simulink model "HEV_Ctrl_V1_1"  (R2018a)
settings: configuration reference "Config_Ctrl" (kept outside this file)
PreLoadFcn:
  | HEV_Ctrl_V1_PreLoad
undefined symbols (not defined in the file or in its folder): AstEnblEngSpdMin_H_K, AstEnblEngSpdMin_L_K, AstEnblSocMin_H_K, AstEnblSocMin_L_K, AstEnblVehSpdMin_H_K, AstEnblVehSpdMin_L_K, AstTrqCmpSOC_K2, AstTrqCmpSOC_X, AstTrqDstBase_K3, DifferentialGearRatio_K, DrvReqPropTrq_K3, DrvReqPropTrqMax_K, eHevCtrlMode, EngTrqMax_K2, EngTrqMax_K2x, HevCtrlEnbl_K, RchEnblEngSpdMin_H_K, RchEnblEngSpdMin_L_K, RchgEnblSocMax_H_K, RchgEnblSocMax_L_K, RchgTrqCmpSOC_K2, RchgTrqCmpSOC_X, RegnBrkCmpSOC_K2, RegnBrkCmpSOC_X, RegnBrkEnblBrkPdlMin_H_K, RegnBrkEnblBrkPdlMin_L_K, RegnBrkEnblSocMax_H_K, RegnBrkEnblSocMax_L_K, RegnBrkEnblVehSpdMin_H_K, RegnBrkEnblVehSpdMin_L_K, TransmissionGearRatio_K2
libraries: simulink x1
(part 2 of 2)

== stateflow chart HEV_Ctrl_V1_1/Hev Control/Energy Management/HevCtrlModeChart ==
  state HEV_control_mode
    state RegnBrake
      en:
      RegnBrk_event;
      HevCtrlMode = RegenBrake;
    state Assist
      en:
      Assist_event;
      HevCtrlMode = Assist;
    state ChargeBattery
      en:
      Rchg_event;
      HevCtrlMode = ReCharge;
    state EngineStart
      en:
      EngStart_event;
      HevCtrlMode = EngineStart;
    state MotorStandby
      en:
      Stby_event;
      HevCtrlMode = Standby;
    (default) -> (junction 3)
    HEV_control_mode -> (junction 3)
    (junction 3) -> RegnBrake [order 1] : [RegnBrkReq]
    (junction 3) -> (junction 9) [order 2]
    (junction 9) -> Assist [order 1] : [MtrAstReq]
    (junction 9) -> (junction 12) [order 2]
    (junction 12) -> ChargeBattery [order 1] : [RchgDrvReq]
    (junction 12) -> (junction 30) [order 2]
    (junction 30) -> EngineStart [order 1] : [EngStartReq]
    (junction 30) -> (junction 15) [order 2]
    (junction 15) -> MotorStandby
  data: RegnBrkReq input; HevCtrlMode output Enum: eHevCtrlMode; MtrAstReq input; RchgDrvReq input; EngStartReq input
  events: RegnBrk_event output FUNCTION_CALL_EVENT; Assist_event output FUNCTION_CALL_EVENT; Rchg_event output FUNCTION_CALL_EVENT; EngStart_event output FUNCTION_CALL_EVENT; Stby_event output FUNCTION_CALL_EVENT

== stateflow chart HEV_Ctrl_V1_1/Task_Schedular/Task_Schedular_Chart ==
  state Control_Task_Event_Generator
    state Task20ms [parallel]
      settings: executionOrder=1
      Task20ms -> (junction 7) : every(2,tick)
      (junction 7) -> (junction 11) : {Evnt20ms;}
    Control_Task_Event_Generator -> (junction 9) : {Evnt10ms;}
  (default) -> Control_Task_Event_Generator
  events: Evnt10ms output FUNCTION_CALL_EVENT; Evnt20ms output FUNCTION_CALL_EVENT
